simulink model "tes"  (R2024a)
settings: Solver=VariableStepAuto  StartTime=0.0  StopTime=0.5  RelTol=1e-3
libraries: spsCurrentMeasurementLib x1, spsDistributedParametersLineLib x1, spsGroundLib x1, spsThreePhaseSeriesRLCLoadLib x1, spsThreePhaseVIMeasurementLib x1, spsThreePhaseFaultLib x1, spsThreePhaseSourceLib x1, sps_lib x1
settings Model: Creator=EE-106  LastModifiedBy=EE-106

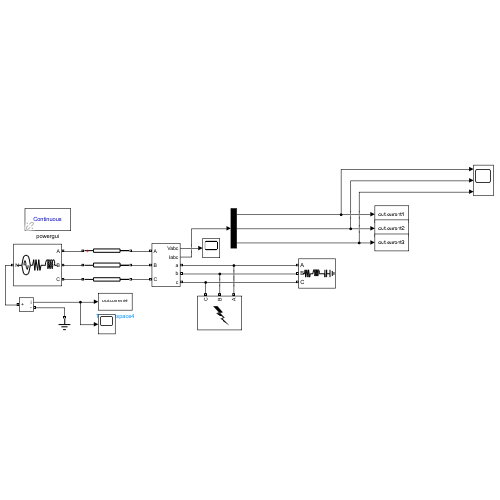
[thumbnail: Simulink's stored preview of the top-level diagram]
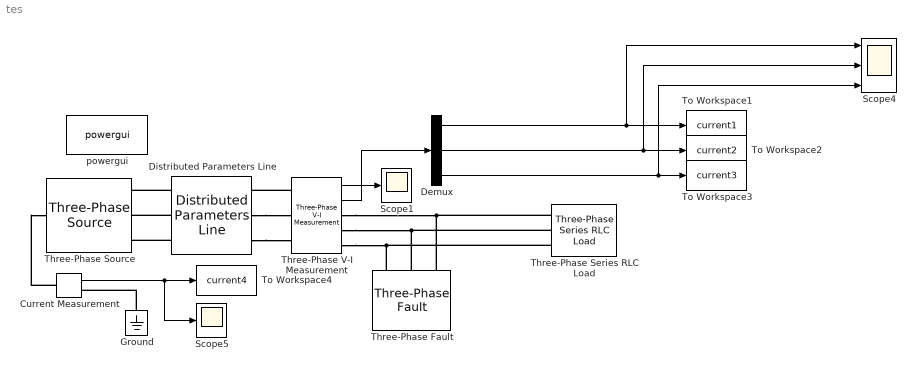
== system tes ==
  Current Measurement : spsCurrentMeasurementLib/Current Measurement  PhasorSimulation=off  OutputType=Complex  PSBequivalent=0
  Demux : Demux  Outputs=3
  Distributed Parameters Line : spsDistributedParametersLineLib/Distributed Parameters Line  Phases=3  Length=100  Frequency=60  Resistance=[0.01273 0.3864]  Inductance="[0.9337e-3  4.1264e-3]"  Capacitance=[12.74e-9 7.751e-9]  x1=[1.62695358267213e-11 24367.5216954237 24367.5216954237;376.991118430775 376.991118430775 376.991118430775;-2.89114919244981 0.34134683233441 -1.22944949446049]  x2=[1.74055996549256e-11 22903.9743931947 22903.9743931947;376.991118430775 376.991118430775 376.991118430775;0.776835825366408 0.00478408175093819 -1.56601224504396]  x3=[1.48933095169727e-13 143.148104219827 143.148104219828;376.991118430775 376.991118430775 376.991118430775;-0.804629671695733 3.01602084032506 1.44522451353016]  x4=[1.88237324433754e-13 312.831121651998 312.831121651999;376.991118430775 376.991118430775 376.991118430775;2.29959221931354 0.00478408175093793 -1.56601224504396]  x5=0.000565541566995742  V1=[1.627e-11 2.437e+04 2.437e+04;377 377 377;-2.891 0.3413 -1.229]  V2=[1.741e-11 2.29e+04 2.29e+04;377 377 377;0.7768 0.004784 -1.566]  I1=[1.489e-13 143.1 143.1;377 377 377;-0.8046 3.016 1.445]  I2=[1.882e-13 312.8 312.8;377 377 377;2.3 0.004784 -1.566]  nHarmo=1  Measurements=None  Decoupling=off  VsMag0=0  VrMag0=0  VsAngle0=0  VrAngle0=0  IsMag0=0  IrMag0=0  IsAngle0=0  IrAngle0=0
      settings: LibrarySourceBlock=sps_lib/Power Grid Elements/Distributed Parameters Line
  Ground : spsGroundLib/Ground  LConnTagsString=a
  Scope1 : Scope
  Scope4 : Scope  NumInputPorts=3
  Scope5 : Scope
  Three-Phase Series RLC Load : spsThreePhaseSeriesRLCLoadLib/Three-Phase Series RLC Load  LConnTagsString=A|B|C  Configuration=Y (grounded)  NominalVoltage=1000  Vabc=[1e3 1e3 1e3]  Vabcp=[1e3 1e3 1e3]  NominalFrequency=60  UnbalancedPower=off  ActivePower=10e3  InductivePower=100  CapacitivePower=100  Pabc=[10e3 9e3 11e3]  QLabc=[100 90 110]  QCabc=[100 90 110]  Pabcp=[10e3 9e3 11e3]  QLabcp=[100 90 110]  QCabcp=[100 90 110]  Measurements=None  LoadType=constant Z
  Three-Phase V-I Measurement : spsThreePhaseVIMeasurementLib/Three-Phase V-I Measurement  VoltageMeasurement=phase-to-ground  SetLabelV=off  LabelV=Vabc  Vpu=on  VpuLL=off  CurrentMeasurement=yes  SetLabelI=off  LabelI=Iabc  Ipu=on  Pbase=500e3  Vbase=100e6  OutputType=Complex  PhasorSimulation=off  PSBequivalent=0
  Three-Phase Fault : spsThreePhaseFaultLib/Three-Phase Fault  InitialStates=0  FaultA=on  FaultB=on  FaultC=off  GroundFault=on  SwitchTimes="[10/60  20/60]"  External=off  SwitchStatus=NaN  FaultResistance=0.0001  GroundResistance=0.01  SnubberResistance=1e6  SnubberCapacitance=inf  Measurements=None
  Three-Phase Source : spsThreePhaseSourceLib/Three-Phase Source  InternalConnection=Yn  VoltagePhases=off  Voltage=25e3  PhaseAngle=0  Voltage_phases=[25e3 25e3 25e3]/sqrt(3)  PhaseAngles_phases=[0 -120 +120]  Frequency=60  NonIdealSource=on  SpecifyImpedance=off  Resistance=0.8929  Inductance=16.58e-3  ShortCircuitLevel=100e6  BaseVoltage=25e3  XRratio=7  BusType=PV  Pref=10e3  Qref=0  Prefabc=[10e3, 10e3, 10e3]  Qrefabc=[0, 0, 0]  Qmin=-inf  Qmax=inf
  To Workspace1 : ToWorkspace  VariableName=current1  SampleTime=-1
  To Workspace2 : ToWorkspace  VariableName=current2  SampleTime=-1
  To Workspace3 : ToWorkspace  VariableName=current3  SampleTime=-1
  To Workspace4 : ToWorkspace  VariableName=current4  SampleTime=-1
  powergui : sps_lib/powergui  Priority=1  SimulationMode=Continuous  SampleTime=5e-05  frequency=60  Iterations=50  frequencyindice=60  Pbase=100e6  ErrMax=1e-4  UnitsV=kV  UnitsW=MW  buscounter=0  FunctionMessages=off  echomessages=off  EnableUseOfTLC=off  CurrentSourceSwitches=off  DisableSnubberDevices=off  DisableRonSwitches=off  DisableVfSwitches=off  DisplayEquations=off  AutomaticDiscreteSolvers=off  SolverType=Tustin/Backward Euler (TBE)  Interpol=off  ExternalGateDelay=off  methode=off  Ts=100  x0status=blocks  SPID=on  SwTol=0  HookPort=off  NonlinearTolerance=1e-4  nMaxIteration=100  ContinueOnMaxIteration=off  RestoreLinks=warning  ResistiveCurrentMeasurement=off  Frange=[0:2:500]  Ylog=off  Xlog=on  ShowGrid=off  save=off  variable=ZData  structure=0  ZoomFFT=off  StartTime=0.0  cycles=1  DisplayStyle=1  fundamental=60  FreqAxis=off  MaxFrequency=1000  frequencyindicesteady=1  RmsSteady=1  display=off
  wires:
  Demux/1 -> Scope4/1, To Workspace1/1
  Demux/2 -> Scope4/2, To Workspace2/1
  Demux/3 -> Scope4/3, To Workspace3/1
  Three-Phase V-I Measurement/1 -> Scope1/1
  Three-Phase V-I Measurement/2 -> Demux/1
  Current Measurement/1 -> Scope5/1, To Workspace4/1
  connections:
  Distributed Parameters Line/LConn1 -- Three-Phase Source/RConn1
  Distributed Parameters Line/LConn2 -- Three-Phase Source/RConn2
  Distributed Parameters Line/LConn3 -- Three-Phase Source/RConn3
  Three-Phase V-I Measurement/LConn1 -- Distributed Parameters Line/RConn1
  Distributed Parameters Line/RConn2 -- Three-Phase V-I Measurement/LConn2
  Distributed Parameters Line/RConn3 -- Three-Phase V-I Measurement/LConn3
  Three-Phase V-I Measurement/RConn1 -- Three-Phase Series RLC Load/LConn1 -- Three-Phase Fault/LConn1
  Three-Phase V-I Measurement/RConn2 -- Three-Phase Fault/LConn2 -- Three-Phase Series RLC Load/LConn2
  Three-Phase V-I Measurement/RConn3 -- Three-Phase Series RLC Load/LConn3 -- Three-Phase Fault/LConn3
  Ground/LConn1 -- Current Measurement/RConn1
  Current Measurement/LConn1 -- Three-Phase Source/LConn1
